simulink model "State_Actions"  (R2025b)
settings: Solver=FixedStepDiscrete  StartTime=0.0  StopTime=10.0  FixedStep=0.01  RelTol=1e-3
libraries: simulink x1
settings Model: Creator=soura  LastModifiedBy=soura

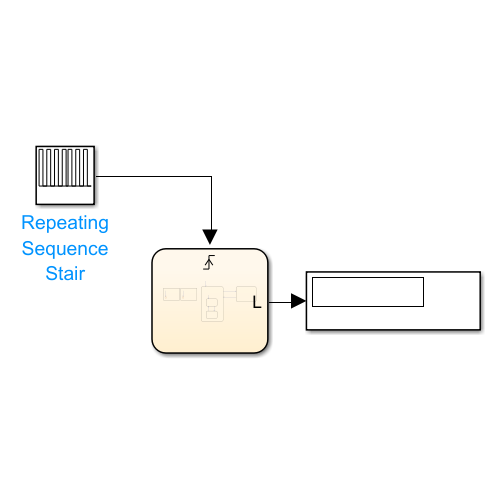
[thumbnail: Simulink's stored preview of the top-level diagram]
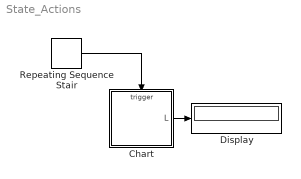
== system State_Actions ==
  Chart : Stateflow chart  TreatAsAtomicUnit=on
  Display : Display
  Repeating Sequence Stair : simulink/Sources/Repeating Sequence Stair  OutValues=[1 0 1 0 1 0 1 0 1 0 1 0 1 0].'  tsamp=-1  OutMin=[]  OutMax=[]  OutDataTypeStr=fixdt('boolean')  OutputDataTypeScalingMode=Specify via dialog  OutDataType=fixdt('boolean')  ConRadixGroup=Best Precision: Vector-wise  OutScaling=[]
  wires:
  Repeating Sequence Stair/1 -> Chart/Trigger
  Chart/1(L) -> Display/1

== stateflow chart State_Actions/Chart ==
  settings: executeAtInitialization=1
  note: Control Chart Execution by Using Temporal Logic - MATLAB & Simulink
  state A1
    en: L=1;
    ex: L=3;
    bind: K;
    state On
      du:L=6;
      send (K)
    state Off
      du:L=11;
    (default) -> On
    Off -> On : [L==11]
    On -> Off : K
  state B1
    on msg: L=5;
    on E:event();
    ex: L=4;
  state event [function]
    (default) -> (junction 27) : {send(msg)}
  (default) -> A1
  A1 -> B1 : at(3,E)
  B1 -> A1 : [L==5]
  data: L output; msg local double =0
  events: E input RISING_EDGE_EVENT; K local FUNCTION_CALL_EVENT
